simulink model "Ass2_System_Open"  (Simulink 8.2)
settings: Solver=ode45  SolverMode=SingleTasking  StartTime=0.0  StopTime=T  RelTol=1e-6  AbsTol=1e-9
settings Model: Creator=schuurmans  LastModifiedBy=yuanyang
settings DataIOCC: LimitDataPoints=off
settings OptimizationCC: BooleanDataType=off  InitFltsAndDblsToZero=on
settings DebuggingCC: SaveWithParameterizedLinksMsg=none  SignalResolutionControl=TryResolveAllWithWarning  SolverPrmCheckMsg=none  MultiTaskDSMMsg=warning  MultiTaskCondExecSysMsg=none
settings HardwareCC: TargetUnknown=on
settings RTWCC: IncludeERTFirstTime=on
settings CodeAppCC: IgnoreCustomStorageClasses=off
settings GRTTargetCC: TargetFcnLib=ansi_tfl_tmw.mat  ModelReferenceCompliant=off  MatFileLogging=off

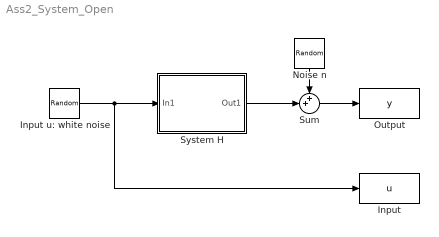
== system Ass2_System_Open ==
  Input : ToWorkspace  VariableName=u  SampleTime=0.01
  Input u: white noise : RandomNumber  Variance=0.5  Seed=1243  SampleTime=0
  Noise n : RandomNumber  Variance=0.1  Seed=876348  SampleTime=0
  Output : ToWorkspace  VariableName=y  SampleTime=0.01
  Sum : Sum  Inputs=++|  SaturateOnIntegerOverflow=on  InputSameDT=on  OutDataTypeStr=Inherit: Same as first input
  System H : Subsystem
  wires:
  Input u: white noise/1 -> System H/1(In1), Input/1
  Noise n/1 -> Sum/1
  System H/1(Out1) -> Sum/2
  Sum/1 -> Output/1

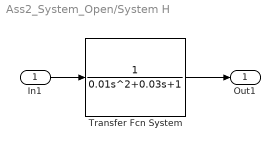
== system Ass2_System_Open/System H ==
  In1 : Inport
  Transfer Fcn System : TransferFcn  Numerator=1  Denominator=[0.01 0.03 1]
  Out1 : Outport  InitialOutput=0
  wires:
  In1/1 -> Transfer Fcn System/1
  Transfer Fcn System/1 -> Out1/1
